simulink model "test1"  (R2022b)
settings: Solver=VariableStepAuto  StartTime=0.0  StopTime=10.0  RelTol=1e-3
libraries: shared6dof x1, sharedtransform x1
settings Model: Creator=User  LastModifiedBy=User

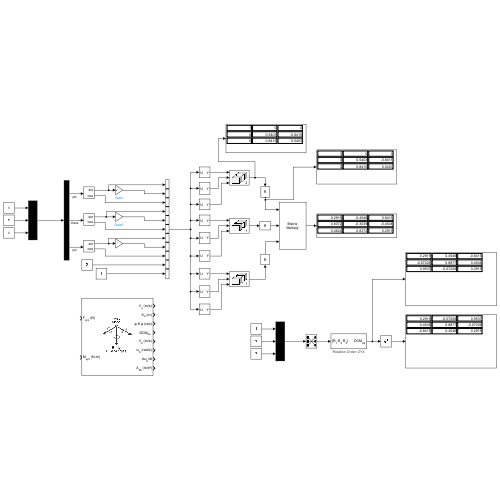
[thumbnail: Simulink's stored preview of the top-level diagram]
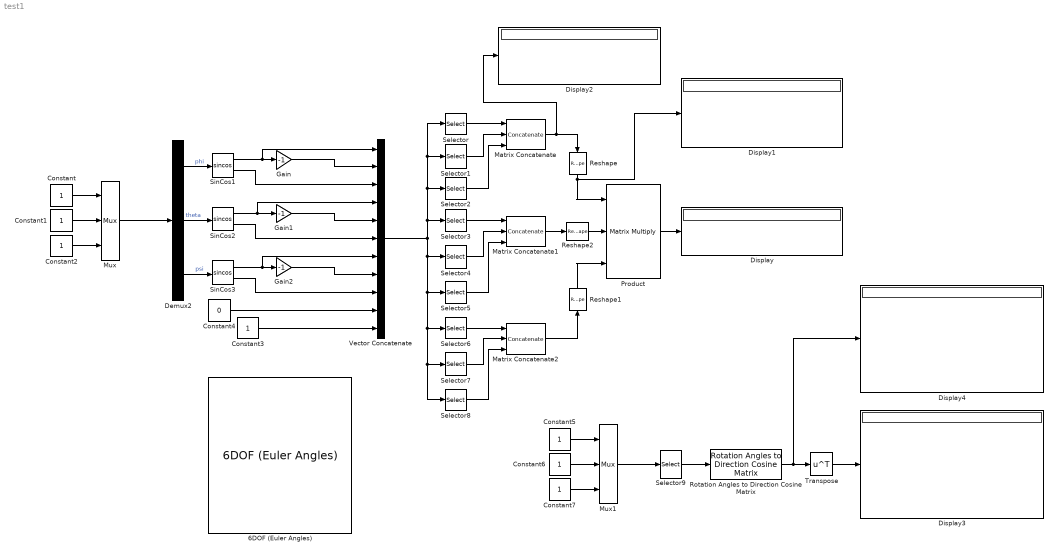
== system test1 ==
  6DOF (Euler Angles) : shared6dof/6DOF (Euler Angles)  units=Metric (MKS)  mtype=Fixed  rep=Euler Angles  xme_0=[0 0 0]  Vm_0=[0 0 0]  eul_0=[0 0 0]  pm_0=[0 0 0]  mass_0=1.0  mass_e=0.5  mass_f=2.0  inertia=eye(3)  inertia_e=eye(3)  inertia_f=2*eye(3)  k_quat=1.0  vre_flag=on  abi_flag=off  aMode=0  xme_statename=''  Vm_statename=''  eul_statename=''  quat_statename=''  pm_statename=''  mass_statename=''
  Constant{,1..3,5..7} (7 alike) : Constant
  Constant4 : Constant  Value=0
  Demux2 : Demux  Outputs=3
  Display{,1..4} (5 alike) : Display
  Gain : Gain  Gain=-1
  Gain1 : Gain  Gain=-1
  Gain2 : Gain  Gain=-1
  Matrix Concatenate : Concatenate  NumInputs=3  Mode=Multidimensional array  ConcatenateDimension=2
  Matrix Concatenate1 : Concatenate  NumInputs=3  Mode=Multidimensional array
  Matrix Concatenate2 : Concatenate  NumInputs=3  Mode=Multidimensional array
  Mux : Mux  Inputs=3
  Mux1 : Mux  Inputs=3
  Product : Product  Inputs=3  Multiplication=Matrix(*)
  Reshape : Reshape  OutputDimensionality=Customize  OutputDimensions=[3,3]
  Reshape1 : Reshape  OutputDimensionality=Customize  OutputDimensions=[3,3]
  Reshape2 : Reshape  OutputDimensionality=Customize  OutputDimensions=[3,3]
  Rotation Angles to Direction Cosine Matrix : sharedtransform/Rotation Angles to Direction Cosine Matrix  rotationOrder=ZYX  aMode=aMode
  Selector : Selector  InputPortWidth=11  IndexOptions=Index vector (dialog)  Indices=[11 10 10]  OutputSizes=1
  Selector1 : Selector  InputPortWidth=11  IndexOptions=Index vector (dialog)  Indices=[10 3 1]  OutputSizes=1
  Selector2 : Selector  InputPortWidth=11  IndexOptions=Index vector (dialog)  Indices=[10 2 3]  OutputSizes=1
  Selector3 : Selector  InputPortWidth=11  IndexOptions=Index vector (dialog)  Indices=[6 10 5]  OutputSizes=1
  Selector4 : Selector  InputPortWidth=11  IndexOptions=Index vector (dialog)  Indices=[10 11 10]  OutputSizes=1
  Selector5 : Selector  InputPortWidth=11  IndexOptions=Index vector (dialog)  Indices=[4 10 6]  OutputSizes=1
  Selector6 : Selector  InputPortWidth=11  IndexOptions=Index vector (dialog)  Indices=[9 7 10]  OutputSizes=1
  Selector7 : Selector  InputPortWidth=11  IndexOptions=Index vector (dialog)  Indices=[8 9 10]  OutputSizes=1
  Selector8 : Selector  InputPortWidth=11  IndexOptions=Index vector (dialog)  Indices=[10 10 11]  OutputSizes=1
  Selector9 : Selector  InputPortWidth=3  IndexOptions=Index vector (dialog)  Indices=[3 2 1]  OutputSizes=1
  SinCos1 : Trigonometry  Operator=sincos
  SinCos2 : Trigonometry  Operator=sincos
  SinCos3 : Trigonometry  Operator=sincos
  Transpose : Math  Operator=transpose
  Vector Concatenate : Concatenate  NumInputs=11
  wires:
  Demux2/3 -> SinCos3/1  "psi"
  Demux2/2 -> SinCos2/1  "theta"
  Vector Concatenate/1 -> Selector/1, Selector1/1, Selector2/1, Selector3/1, Selector6/1, Selector8/1, Selector7/1, Selector5/1, Selector4/1
  Demux2/1 -> SinCos1/1  "phi"
  Mux/1 -> Demux2/1
  Selector/1 -> Matrix Concatenate/1
  Selector1/1 -> Matrix Concatenate/2
  Selector2/1 -> Matrix Concatenate/3
  Constant/1 -> Mux/1
  Constant1/1 -> Mux/2
  Constant2/1 -> Mux/3
  SinCos1/1 -> Vector Concatenate/1, Gain/1
  Gain/1 -> Vector Concatenate/2
  SinCos1/2 -> Vector Concatenate/3
  SinCos2/1 -> Vector Concatenate/4, Gain1/1
  Gain1/1 -> Vector Concatenate/5
  SinCos2/2 -> Vector Concatenate/6
  SinCos3/1 -> Vector Concatenate/7, Gain2/1
  Gain2/1 -> Vector Concatenate/8
  SinCos3/2 -> Vector Concatenate/9
  Constant4/1 -> Vector Concatenate/10
  Constant3/1 -> Vector Concatenate/11
  Selector3/1 -> Matrix Concatenate1/1
  Selector4/1 -> Matrix Concatenate1/2
  Selector5/1 -> Matrix Concatenate1/3
  Selector8/1 -> Matrix Concatenate2/3
  Selector7/1 -> Matrix Concatenate2/2
  Selector6/1 -> Matrix Concatenate2/1
  Matrix Concatenate/1 -> Display2/1, Reshape/1
  Matrix Concatenate1/1 -> Reshape2/1
  Matrix Concatenate2/1 -> Reshape1/1
  Reshape/1 -> Product/1, Display1/1
  Reshape2/1 -> Product/2
  Reshape1/1 -> Product/3
  Product/1 -> Display/1
  Constant7/1 -> Mux1/3
  Constant6/1 -> Mux1/2
  Constant5/1 -> Mux1/1
  Mux1/1 -> Selector9/1
  Selector9/1 -> Rotation Angles to Direction Cosine Matrix/1
  Rotation Angles to Direction Cosine Matrix/1 -> Display4/1, Transpose/1
  Transpose/1 -> Display3/1
